simulink model "F16_2003hiModelAutopilot_steadySim"  (R2013a)
settings: Solver=ode3  StartTime=0.0  StopTime=100  FixedStep=0.01  RelTol=1e-5
values from neighbouring files (symbols this model uses):
  A = [0	0	0	0	0	0	1	0	0	0	0	0	0	0	0	0	0	0 ... (first row only)    [F16NolinearModelRemoveWindControlData_low.m]    (also in F16_2003hiModelAutopilot.m = [0	0	0	0	-2.55E-09	0	1	0	0	0	0	0	0	0	0	0	0	0; F16_2003hiModelAutopilot1.m = [0	0	0	0	-2.55E-09	0	1	0	0	0	0	0	0	0	0	0	0	0; F16_2003hiModelAutopilot1_steadySys.m = [0	0	0	0	-2.55E-09	0	1	0	0	0	0	0	0	0	0	0	0	0; LQR_Calc2.m = [A1,zeros(8,2);-C_v_theta,zeros(2,2)])
  A_la = A([2,4,6,9,10,12,15,16],[2,4,6,9,10,12,15,16])    [F16NolinearModelRemoveWindControlData_low.m]    (also in F16_2003hiModelAutopilot.m; F16_2003hiModelAutopilot1.m; F16_2003hiModelAutopilot1_steadySys.m = A([4,6,9,10,12,15,16],[4,6,9,10,12,15,16]); LQR_Calc2_F16YingHu_lonAndLa.m = A_full(8:12,8:12))
  A_lon = A([1,3,5,7,8,11,13,14],[1,3,5,7,8,11,13,14])    [F16NolinearModelRemoveWindControlData_low.m]    (also in F16_2003hiModelAutopilot.m; F16_2003hiModelAutopilot1.m; F16_2003hiModelAutopilot1_steadySys.m = A([5,7,8,11,13,14],[5,7,8,11,13,14]); LQR_Calc2_F16YingHu_lonAndLa.m = A_full(1:7,1:7))
  B = [0	0	0	0 ... (first row only)    [F16NolinearModelRemoveWindControlData_low.m]    (also in F16_2003hiModelAutopilot.m; F16_2003hiModelAutopilot1.m; F16_2003hiModelAutopilot1_steadySys.m; LQR_Calc2.m = [B1;zeros(2,2)])
  B_la = B([2,4,6,9,10,12,15,16],3:4)    [F16NolinearModelRemoveWindControlData_low.m]    (also in F16_2003hiModelAutopilot.m; F16_2003hiModelAutopilot1.m; F16_2003hiModelAutopilot1_steadySys.m = B([4,6,9,10,12,15,16],3:4); LQR_Calc2_F16YingHu_lonAndLa.m = B_full(8:12,3:4))
  B_lon = B([1,3,5,7,8,11,13,14],1:2)    [F16NolinearModelRemoveWindControlData_low.m]    (also in F16_2003hiModelAutopilot.m; F16_2003hiModelAutopilot1.m; F16_2003hiModelAutopilot1_steadySys.m = B([5,7,8,11,13,14],1:2); LQR_Calc2_F16YingHu_lonAndLa.m = B_full(1:7,1:2))
  Kp = zeros(4,18)    [F16NolinearModelRemoveWindControlData_low.m]    (also in F16_2003hiModelAutopilot.m; F16_2003hiModelAutopilot1.m; F16_2003hiModelAutopilot1_steadySys.m; LQR_Calc2.m = k(:,1:8))
  Kp_la = k_la(:,1:8)    [F16NolinearModelRemoveWindControlData_low.m]    (also in F16_2003hiModelAutopilot.m; F16_2003hiModelAutopilot1.m; F16_2003hiModelAutopilot1_steadySys.m = k_la; LQR_Calc2_F16YingHu_lonAndLa.m = k_la(:,1:5))
undefined symbols (not defined in the file or in its folder): k_lon
settings Model: Creator=Dai  LastModifiedBy=Dai

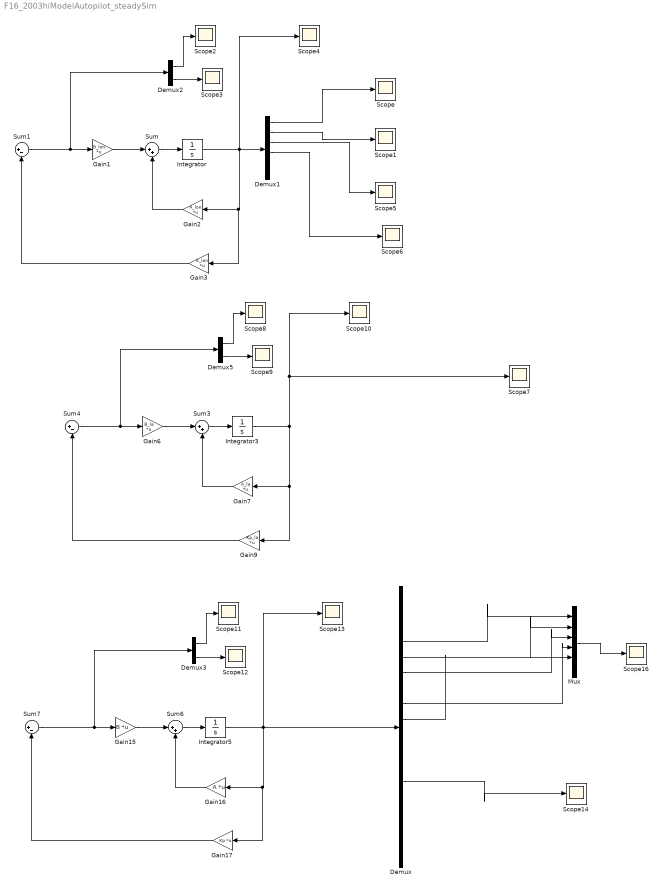
== system F16_2003hiModelAutopilot_steadySim ==
  Demux : Demux  Outputs=18
  Demux1 : Demux  Outputs=6
  Demux2 : Demux  Outputs=2
  Demux3 : Demux  Outputs=2
  Demux5 : Demux  Outputs=2
  Gain1 : Gain  Gain=B_lon  Multiplication=Matrix(K*u) (u vector)
  Gain15 : Gain  Gain=B  Multiplication=Matrix(K*u) (u vector)
  Gain16 : Gain  Gain=A  Multiplication=Matrix(K*u) (u vector)
  Gain17 : Gain  Gain=Kp  Multiplication=Matrix(K*u) (u vector)
  Gain2 : Gain  Gain=A_lon  Multiplication=Matrix(K*u) (u vector)
  Gain3 : Gain  Gain=k_lon  Multiplication=Matrix(K*u) (u vector)
  Gain6 : Gain  Gain=B_la  Multiplication=Matrix(K*u) (u vector)
  Gain7 : Gain  Gain=A_la  Multiplication=Matrix(K*u) (u vector)
  Gain9 : Gain  Gain=Kp_la  Multiplication=Matrix(K*u) (u vector)
  Integrator : Integrator  InitialCondition=[0.1,0.1,0.1,0.1,0,0]
  Integrator3 : Integrator  InitialCondition=[0.1,0.1,0.1,0.1,0.1,0,0]
  Integrator5 : Integrator  InitialCondition=[0.1,0.1,0.1,0.1,0.1,0.1,zeros(1,12)]
  Mux : Mux  Inputs=6
  Scope{,1..14,16} (16 alike) : Scope
      Scope10 settings: SaveName=ScopeData9
      Scope11 settings: SaveName=ScopeData15
      Scope12 settings: SaveName=ScopeData16
      Scope13 settings: SaveName=ScopeData11
      Scope14 settings: SaveName=ScopeData13
      Scope16 settings: SaveName=ScopeData12
      Scope2 settings: SaveName=ScopeData2
      Scope3 settings: SaveName=ScopeData3
      Scope4 settings: SaveName=ScopeData4
      Scope5 settings: SaveName=ScopeData5
      Scope6 settings: SaveName=ScopeData6
      Scope7 settings: SaveName=ScopeData10
      Scope8 settings: SaveName=ScopeData7
      Scope9 settings: SaveName=ScopeData8
  Sum : Sum  Inputs=|++
  Sum1 : Sum  Inputs=|+-
  Sum3 : Sum  Inputs=|++
  Sum4 : Sum  Inputs=|+-
  Sum6 : Sum  Inputs=|++
  Sum7 : Sum  Inputs=|+-
  wires:
  Integrator/1 -> Demux1/1, Scope4/1, Gain3/1, Gain2/1
  Gain1/1 -> Sum/1
  Sum/1 -> Integrator/1
  Gain2/1 -> Sum/2
  Sum1/1 -> Demux2/1, Gain1/1
  Gain3/1 -> Sum1/2
  Demux2/1 -> Scope2/1
  Demux2/2 -> Scope3/1
  Demux1/1 -> Scope/1
  Demux1/2 -> Scope1/1
  Demux1/3 -> Scope5/1
  Demux1/4 -> Scope6/1
  Integrator3/1 -> Scope7/1, Scope10/1, Gain9/1, Gain7/1
  Gain6/1 -> Sum3/1
  Sum3/1 -> Integrator3/1
  Gain7/1 -> Sum3/2
  Sum4/1 -> Demux5/1, Gain6/1
  Gain9/1 -> Sum4/2
  Demux5/1 -> Scope8/1
  Demux5/2 -> Scope9/1
  Gain15/1 -> Sum6/1
  Sum6/1 -> Integrator5/1
  Gain16/1 -> Sum6/2
  Sum7/1 -> Demux3/1, Gain15/1
  Gain17/1 -> Sum7/2
  Demux3/1 -> Scope11/1
  Demux3/2 -> Scope12/1
  Integrator5/1 -> Demux/1, Scope13/1, Gain17/1, Gain16/1
  Demux/4 -> Mux/1
  Demux/5 -> Mux/2
  Demux/6 -> Mux/3
  Demux/8 -> Mux/4
  Demux/9 -> Mux/5
  Mux/1 -> Scope16/1
  Demux/13 -> Scope14/1
